simulink model "threeD_mod5_Counter"  (R2020a)
settings: Solver=VariableStepAuto  StartTime=0.0  StopTime=10.0  RelTol=1e-3
settings Model: Creator=INDRAJIT MARATHE  LastModifiedBy=INDRAJIT MARATHE

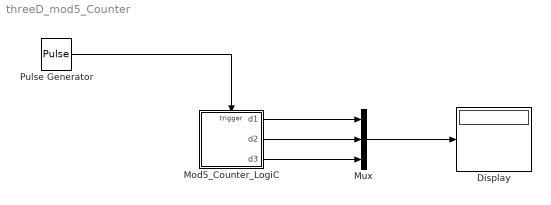
== system threeD_mod5_Counter ==
  "Display " : Display
  Mod5_Counter_LogiC : Stateflow chart  TreatAsAtomicUnit=on
  Mux : Mux  Inputs=3
  "Pulse Generator " : DiscretePulseGenerator  PulseType=Time based  Period=0.1  PulseWidth=50
  wires:
  Mux/1 -> "Display "/1
  Mod5_Counter_LogiC/2(d2) -> Mux/2
  Mod5_Counter_LogiC/1(d1) -> Mux/1
  Mod5_Counter_LogiC/3(d3) -> Mux/3
  "Pulse Generator "/1 -> Mod5_Counter_LogiC/Trigger

== stateflow chart threeD_mod5_Counter/Mod5_Counter_LogiC ==
  state digit1 [parallel]
    settings: executionOrder=1
    state Zero
      en: d1= 0;
    state One
      en: d1= 1;
    state Three
      en: d1= 3;
    state Two
      en:d1=2;
    state Four
      en:d1=4;
    (default) -> digit1.Zero
    digit1.Zero -> digit1.One : inc1
    digit1.One -> digit1.Two : inc1
    digit1.Two -> digit1.Three : inc1
    digit1.Three -> digit1.Four : inc1
    digit1.Four -> digit1.Zero : inc1/{inc2}
  state digit2 [parallel]
    settings: executionOrder=2
    state Zero
      en: d2= 0;
    state One
      en: d2= 1;
    state Four
      en: d2= 4;
    state Two
      en:d2=2;
    state Three
      en:d2=3;
    (default) -> digit2.Zero
    digit2.Zero -> digit2.One : inc2
    digit2.One -> digit2.Two : inc2
    digit2.Two -> digit2.Three : inc2
    digit2.Three -> digit2.Four : inc2
    digit2.Four -> digit2.Zero : inc2/{inc3}
  state digit3 [parallel]
    settings: executionOrder=3
    state Zero
      en: d3= 0;
    state One
      en: d3= 1;
    state Two
      en: d3= 2;
    state Three
      en: d3= 3;
    state Four
      en: d3= 4;
    (default) -> digit3.Zero
    digit3.Zero -> digit3.One : inc3
    digit3.One -> digit3.Two : inc3
    digit3.Two -> digit3.Three : inc3
    digit3.Three -> digit3.Four : inc3
    digit3.Four -> digit3.Zero : inc3
  data: d1 output; d2 output; d3 output
  events: inc1 input RISING_EDGE_EVENT; inc2 input RISING_EDGE_EVENT; inc3 input RISING_EDGE_EVENT
